simulink model "L1_ent"  (Simulink 7.0)
settings: Solver=ode45  StartTime=0.0  StopTime=90  RelTol=1e-7
values from neighbouring files (symbols this model uses):
  K1 = 1    [Systementkopplung_ini.m]
  K2 = 7    [Systementkopplung_ini.m]
  K3 = 6    [Systementkopplung_ini.m]
  K4 = 5    [Systementkopplung_ini.m]
  K5 = 4    [Systementkopplung_ini.m]
  K6 = 1.5    [Systementkopplung_ini.m]
  K7 = 2    [Systementkopplung_ini.m]
  K8 = 1    [Systementkopplung_ini.m]
  T1 = 1    [Systementkopplung_ini.m]
  T3 = 2    [Systementkopplung_ini.m]
  T4 = 2.5    [Systementkopplung_ini.m]
  T5 = 3    [Systementkopplung_ini.m]
  T6 = 3.5    [Systementkopplung_ini.m]
  T7 = 4    [Systementkopplung_ini.m]
Description:
  | 2 gekoppelte Regelstrecken
settings Model: Creator=Sz  LastModifiedBy=psz

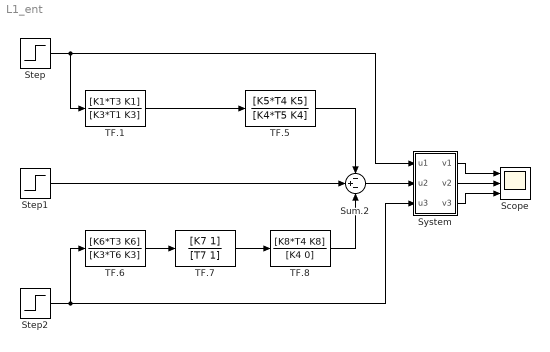
== system L1_ent ==
  Scope : Scope  NumInputPorts=3
      settings: TimeRange=90  YMin=0~-10~0  YMax=250~30~1.5
  Step : Step  Time=60  SampleTime=0
  Step1 : Step  Time=30  SampleTime=0
  Step2 : Step  Time=0  SampleTime=0
  Sum.2 : Sum  Inputs=-+-  OutDataType=sfix(16)  OutScaling=2^0  SaturateOnIntegerOverflow=on  InputSameDT=on
  System : Subsystem
  TF.1 : TransferFcn  Numerator=[K1*T3 K1]  Denominator=[K3*T1 K3]
  TF.5 : TransferFcn  Numerator=[K5*T4 K5]  Denominator=[K4*T5 K4]
  TF.6 : TransferFcn  Numerator=[K6*T3 K6]  Denominator=[K3*T6 K3]
  TF.7 : TransferFcn  Numerator=[K7 1]  Denominator=[T7 1]
  TF.8 : TransferFcn  Numerator=[K8*T4 K8]  Denominator=[K4 0]
  wires:
  System/2(v2) -> Scope/2
  System/3(v3) -> Scope/3
  System/1(v1) -> Scope/1
  Step/1 -> TF.1/1, System/1(u1)
  Sum.2/1 -> System/2(u2)
  Step1/1 -> Sum.2/2
  Step2/1 -> TF.6/1, System/3(u3)
  TF.1/1 -> TF.5/1
  TF.5/1 -> Sum.2/1
  TF.7/1 -> TF.8/1
  TF.6/1 -> TF.7/1
  TF.8/1 -> Sum.2/3

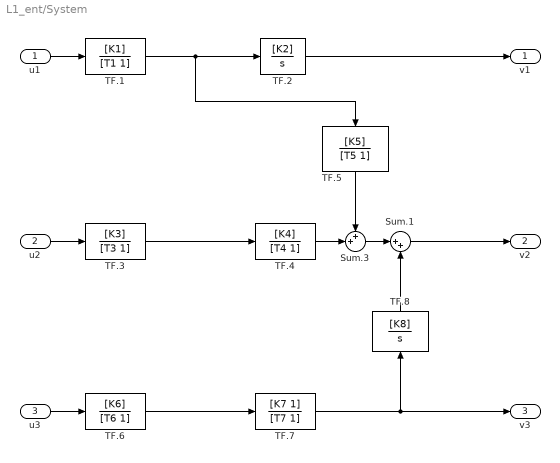
== system L1_ent/System ==
  u1 : Inport
  u2 : Inport  Port=2
  u3 : Inport  Port=3
  Sum.1 : Sum  Inputs=|++  OutDataType=sfix(16)  OutScaling=2^0  SaturateOnIntegerOverflow=on  InputSameDT=on
  Sum.3 : Sum  Inputs=++|  OutDataType=sfix(16)  OutScaling=2^0  SaturateOnIntegerOverflow=on  InputSameDT=on
  TF.1 : TransferFcn  Numerator=[K1]  Denominator=[T1 1]
  TF.2 : TransferFcn  Numerator=[K2]  Denominator=[1 0]
  TF.3 : TransferFcn  Numerator=[K3]  Denominator=[T3 1]
  TF.4 : TransferFcn  Numerator=[K4]  Denominator=[T4 1]
  TF.5 : TransferFcn  Orientation=down  Numerator=[K5]  Denominator=[T5 1]
  TF.6 : TransferFcn  Numerator=[K6]  Denominator=[T6 1]
  TF.7 : TransferFcn  Numerator=[K7 1]  Denominator=[T7 1]
  TF.8 : TransferFcn  Orientation=up  Numerator=[K8]  Denominator=[1 0]
  v1 : Outport
  v2 : Outport  Port=2
  v3 : Outport  Port=3
  wires:
  TF.1/1 -> TF.5/1, TF.2/1
  Sum.1/1 -> v2/1
  Sum.3/1 -> Sum.1/1
  TF.8/1 -> Sum.1/2
  u3/1 -> TF.6/1
  TF.6/1 -> TF.7/1
  TF.7/1 -> TF.8/1, v3/1
  TF.5/1 -> Sum.3/1
  TF.3/1 -> TF.4/1
  u2/1 -> TF.3/1
  u1/1 -> TF.1/1
  TF.4/1 -> Sum.3/2
  TF.2/1 -> v1/1
